simulink model "sdynamics"  (R2020a)
settings: Solver=ode45  StartTime=0.0  StopTime=20000  RelTol=1e-3  EnableMultiTasking=on
PreLoadFcn:
  | clear all
  | path(pathdef)
  | addpath('.')
  | params
InitFcn:
  | clear all
  | path(pathdef)
  | addpath('.')
  | params
StartFcn:
  | clear all
  | path(pathdef)
  | addpath('.')
  | params
undefined symbols (not defined in the file or in its folder): init_states, plots, scraft, scraft_states, sdyn
ContinueFcn:
  | path(pathdef)
  | addpath('.')
  | params
settings Model: NumberOfSteps=1000  Creator=nikhil  LastModifiedBy=VTOL_HYD
settings DataIOCC: LimitDataPoints=on  SaveFormat=Array  SignalLoggingSaveFormat=ModelDataLogs  ReturnWorkspaceOutputs=off
settings OptimizationCC: ExpressionDepthLimit=2147483647  InitFltsAndDblsToZero=on  LifeSpan=inf
settings DebuggingCC: UnderspecifiedInitializationDetection=Classic  MergeDetectMultiDrivingBlocksExec=none  FcnCallInpInsideContextMsg=warning  AllowSymbolicDim=off  StateNameClashWarn=warning  PregeneratedLibrarySubsystemCodeDiagnostic=none  SFUnexpectedBacktrackingDiag=warning  SFNoUnconditionalDefaultTransitionDiag=warning  SFExecutionAtInitializationDiag=none  ArithmeticOperatorsInVariantConditions=warning
settings HardwareCC: ProdBitPerPointer=32  ProdBitPerSizeT=32  ProdBitPerPtrDiffT=32  ProdLargestAtomicFloat=None  ProdIntDivRoundTo=Undefined  ProdEndianess=Unspecified  ProdWordSize=32  ProdHWDeviceType=32-bit Generic
settings ModelReferenceCC: PropagateSignalLabelsOutOfModel=off
settings SFSimCC: SimUseLocalCustomCode=off  CustomCodeUndefinedFunction=UseInterfaceOnly
settings RTWCC: RTWUseLocalCustomCode=off
settings CodeAppCC: StateflowObjectComments=on
settings GRTTargetCC: TargetLangStandard=C89/C90 (ANSI)  CombineOutputUpdateFcns=off  GRTInterface=on
settings ConfigComp: CovMetricSettings=dw  CovHtmlReporting=on  CovSaveCumulativeToWorkspaceVar=on  CovSaveSingleToWorkspaceVar=on  CovExternalEMLEnable=off  CovSFcnEnable=off

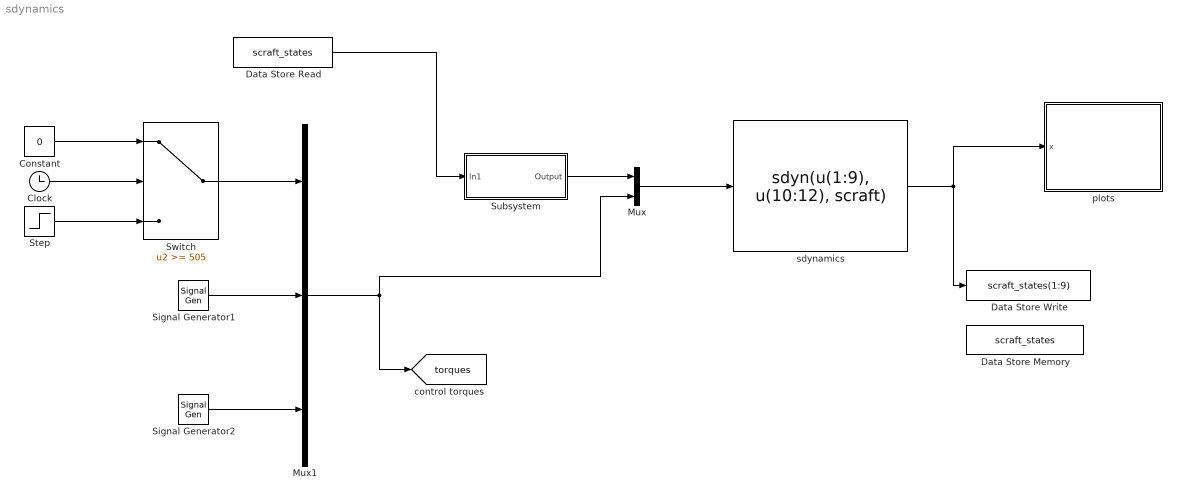
== system sdynamics ==
  Clock : Clock
  Constant : Constant  Value=0  SampleTime=1
  Data Store Memory : DataStoreMemory  LoadFcn=|  InitFcn=|  StartFcn=|  DataStoreName=scraft_states  ReadBeforeWriteMsg=warning  WriteAfterWriteMsg=warning  WriteAfterReadMsg=warning  InitialValue=[0;0;0;0;0;0;0;0;0]  ShowAdditionalParam=off
      | clear all
      | path(pathdef)
      | addpath('.')
      | params
      | clear all
      | path(pathdef)
      | addpath('.')
      | params
      | clear all
      | path(pathdef)
      | addpath('.')
      | params
      settings: ContinueFcn=|
      | clear all
      | path(pathdef)
      | addpath('.')
      | params
  Data Store Read : DataStoreRead  LoadFcn=|  InitFcn=|  StartFcn=|  DataStoreName=scraft_states  SampleTime=1
      | clear all
      | path(pathdef)
      | addpath('.')
      | params
      | clear all
      | path(pathdef)
      | addpath('.')
      | params
      | clear all
      | path(pathdef)
      | addpath('.')
      | params
      settings: ContinueFcn=|
      | clear all
      | path(pathdef)
      | addpath('.')
      | params
  Data Store Write : DataStoreWrite  LoadFcn=|  InitFcn=|  StartFcn=|  DataStoreName=scraft_states  SampleTime=1  DataStoreElements=scraft_states(1:9)
      | clear all
      | path(pathdef)
      | addpath('.')
      | params
      | clear all
      | path(pathdef)
      | addpath('.')
      | params
      | clear all
      | path(pathdef)
      | addpath('.')
      | params
      settings: ContinueFcn=|
      | clear all
      | path(pathdef)
      | addpath('.')
      | params
      settings: OpenFcn=|
      | clear all
      | path(pathdef)
      | addpath('.')
      | params
  Mux : Mux  Inputs=2
  Mux1 : Mux  Inputs=3
  Signal Generator1 : SignalGenerator  Amplitude=0  Units=rad/sec
  Signal Generator2 : SignalGenerator  Amplitude=0  Units=rad/sec
  Step : Step  After=0.01  SampleTime=500
  Subsystem : Subsystem  InitFcn=|
      | clear all
      | path(pathdef)
      | addpath('.')
  Switch : Switch  Threshold=505  ZeroCross=off
  plots : Subsystem  InitFcn=|
      | path(pathdef)
      | addpath('.')
  sdynamics : MATLABFcn  MATLABFcn=sdyn(u(1:9), u(10:12), scraft)  OutputDimensions=9
      mask Display: image(imread('scraft.jpg'))
  tag scope: torques=global
  wires:
  sdynamics/1 -> Data Store Write/1, plots/1(x)
  Mux1/1 -> [torques], Mux/2
  Subsystem/1(Output) -> Mux/1
  Mux/1 -> sdynamics/1
  Switch/1 -> Mux1/1
  Signal Generator1/1 -> Mux1/2
  Signal Generator2/1 -> Mux1/3
  Clock/1 -> Switch/2
  Constant/1 -> Switch/1
  Step/1 -> Switch/3
  Data Store Read/1 -> Subsystem/1(In1)

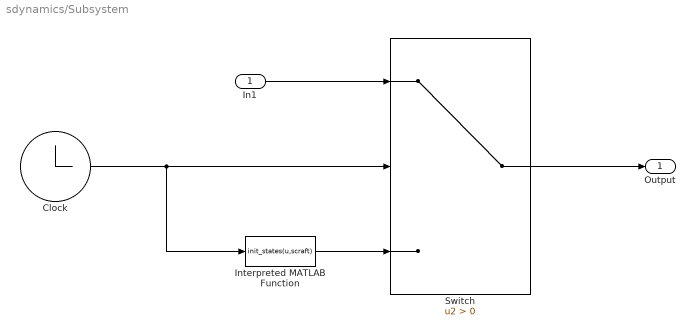
== system sdynamics/Subsystem ==
  In1 : Inport  SampleTime=1
  Clock : Clock
  Interpreted MATLAB Function : MATLABFcn  MATLABFcn=init_states(u,scraft)  OutputDimensions=9
  Switch : Switch  Criteria=u2 > Threshold
  Output : Outport  SampleTime=1  VectorParamsAs1DForOutWhenUnconnected=off
  wires:
  Switch/1 -> Output/1
  In1/1 -> Switch/1
  Interpreted MATLAB Function/1 -> Switch/3
  Clock/1 -> Interpreted MATLAB Function/1, Switch/2

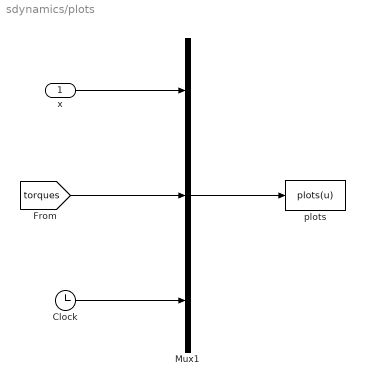
== system sdynamics/plots ==
  x : Inport  SampleTime=1
  Clock : Clock
  Mux1 : Mux  Inputs=3
  plots : MATLABFcn  MATLABFcn=plots(u)  OutputDimensions=0  SampleTime=1
  wires:
  Mux1/1 -> plots/1
  Clock/1 -> Mux1/3
  x/1 -> Mux1/1
  [torques] -> Mux1/2
